simulink model "V3_2_MatlabFn_UnitTest"  (R2017b)
settings: Solver=VariableStepAuto  StartTime=0.0  StopTime=.5  MaxStep=1e-4  RelTol=1e-3
libraries: simulink x9, dspswit3 x1, powerlib x1
settings Model: Creator=Manu Krishnan  LastModifiedBy=Manu Krishnan

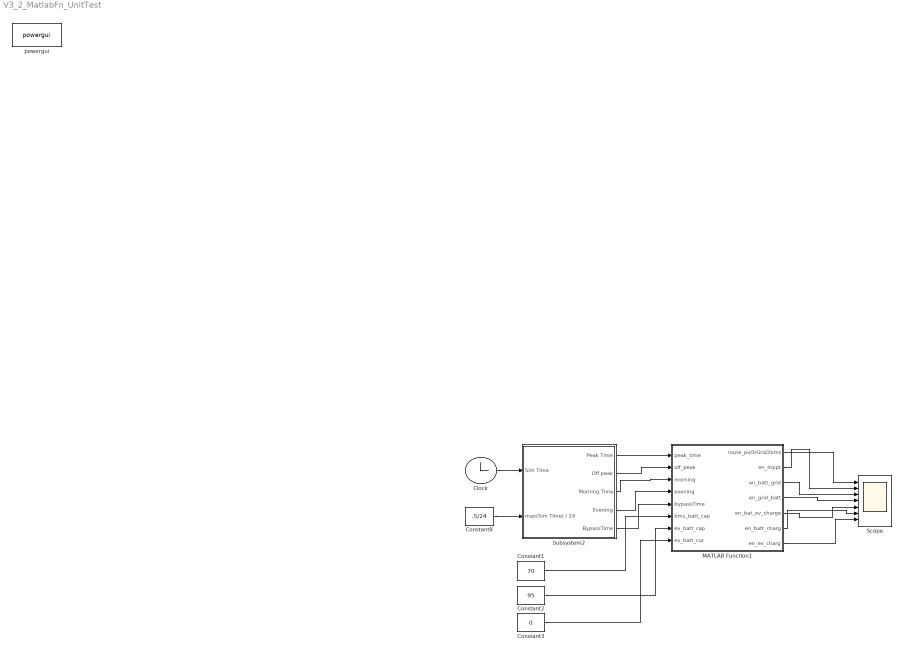
== system V3_2_MatlabFn_UnitTest ==
  Clock : Clock
  Constant1 : Constant  Value=70  VectorParams1D=off
  Constant2 : Constant  Value=95  VectorParams1D=off
  Constant3 : Constant  Value=0  VectorParams1D=off
  Constant8 : Constant  Value=.5/24  VectorParams1D=off
  MATLAB Function1 : MATLAB Function  TreatAsAtomicUnit=on
  Scope : Scope  NumInputPorts=7
  Subsystem2 : Subsystem
  powergui : powerlib/powergui  Priority=1  SimulationMode=Continuous  SampleTime=50e-6  frequency=60  Iterations=50  frequencyindice=0  Pbase=100e6  ErrMax=1e-4  UnitsV=kV  UnitsW=MW  buscounter=0  FunctionMessages=off  echomessages=off  EnableUseOfTLC=off  CurrentSourceSwitches=off  DisableSnubberDevices=off  DisableRonSwitches=off  DisableVfSwitches=off  DisplayEquations=off  SolverType=Tustin/Backward Euler (TBE)  Interpol=off  ExternalGateDelay=off  methode=off  Ts=100  x0status=blocks  SPID=on  SwTol=0  HookPort=off  RestoreLinks=warning  ResistiveCurrentMeasurement=off  Frange=[0:2:500]  Ylog=off  Xlog=on  ShowGrid=off  save=off  variable=ZData  structure=0  ZoomFFT=off  StartTime=0.0  cycles=1  DisplayStyle=1  fundamental=60  FreqAxis=off  MaxFrequency=1000  frequencyindicesteady=1  RmsSteady=1  display=off
  wires:
  Clock/1 -> Subsystem2/1(Sim Time)
  Constant8/1 -> Subsystem2/2(max(Sim Time) / 24)
  Subsystem2/1(Peak Time) -> MATLAB Function1/1(peak_time)
  Subsystem2/2(Off peak) -> MATLAB Function1/2(off_peak)
  Subsystem2/3(Morning Time) -> MATLAB Function1/3(morning)
  Subsystem2/4(Evening) -> MATLAB Function1/4(evening)
  Subsystem2/5(BypassTime) -> MATLAB Function1/5(bypassTime)
  MATLAB Function1/2(en_mppt) -> Scope/2
  MATLAB Function1/3(en_batt_grid) -> Scope/3
  MATLAB Function1/7(en_ev_charg) -> Scope/7
  MATLAB Function1/6(en_batt_charg) -> Scope/6
  MATLAB Function1/1(route_pvOrGrid2bms) -> Scope/1
  MATLAB Function1/5(en_bat_ev_charge) -> Scope/5
  MATLAB Function1/4(en_grid_batt) -> Scope/4
  Constant1/1 -> MATLAB Function1/6(bms_batt_cap)
  Constant2/1 -> MATLAB Function1/7(ev_batt_cap)
  Constant3/1 -> MATLAB Function1/8(ev_batt_cur)

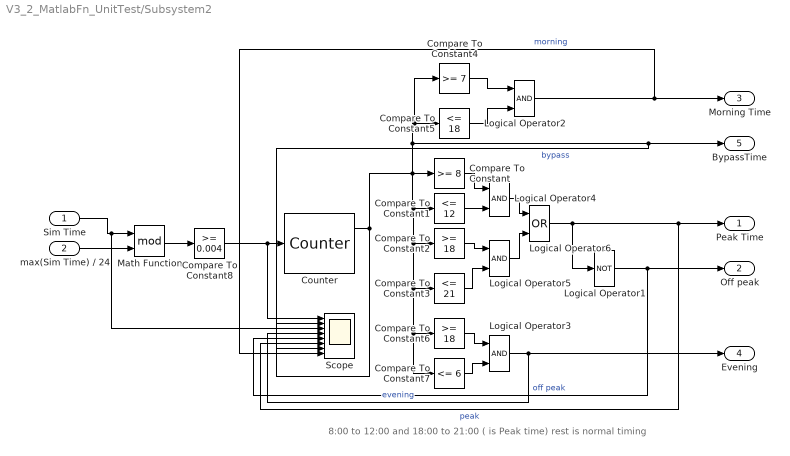
== system V3_2_MatlabFn_UnitTest/Subsystem2 ==
  note: 8:00 to 12:00 and 18:00 to 21:00 ( is Peak time)
      | rest is normal timing
  Sim Time : Inport
  max(Sim Time) / 24 : Inport  Port=2
  Compare To Constant : simulink/Logic and Bit Operations/Compare To Constant  relop=>=  const=8  OutDataTypeStr=boolean  ZeroCross=off
  Compare To Constant1 : simulink/Logic and Bit Operations/Compare To Constant  relop=<=  const=12  OutDataTypeStr=boolean  ZeroCross=off
  Compare To Constant2 : simulink/Logic and Bit Operations/Compare To Constant  relop=>=  const=18  OutDataTypeStr=boolean  ZeroCross=off
  Compare To Constant3 : simulink/Logic and Bit Operations/Compare To Constant  relop=<=  const=21  OutDataTypeStr=boolean  ZeroCross=off
  Compare To Constant4 : simulink/Logic and Bit Operations/Compare To Constant  relop=>=  const=7  OutDataTypeStr=boolean  ZeroCross=off
  Compare To Constant5 : simulink/Logic and Bit Operations/Compare To Constant  relop=<=  const=18  OutDataTypeStr=boolean  ZeroCross=off
  Compare To Constant6 : simulink/Logic and Bit Operations/Compare To Constant  relop=>=  const=18  OutDataTypeStr=boolean  ZeroCross=off
  Compare To Constant7 : simulink/Logic and Bit Operations/Compare To Constant  relop=<=  const=6  OutDataTypeStr=boolean  ZeroCross=off
  Compare To Constant8 : simulink/Logic and Bit Operations/Compare To Constant  relop=>=  const=0.004  OutDataTypeStr=boolean  ZeroCross=off
  Counter : dspswit3/Counter  Direction=Up  CountEvent=Falling edge  CounterSize=User defined  MaxCount=24  InitialCount=0  Output=Count and Hit  HitValue=24  ResetInput=off  SamplesPerFrame=1  Ts=1  CntDtype=int8  HitDtype=Logical
  Logical Operator1 : Logic  Operator=NOT  AllPortsSameDT=off  OutDataTypeStr=boolean
  Logical Operator{2..5} (4 alike) : Logic  AllPortsSameDT=off  OutDataTypeStr=boolean
  Logical Operator6 : Logic  Operator=OR  AllPortsSameDT=off  OutDataTypeStr=boolean
  Math Function : Math  Operator=mod  SaturateOnIntegerOverflow=on
  Scope : Scope  NumInputPorts=8
  Peak Time : Outport
  Off peak : Outport  Port=2
  Morning Time : Outport  Port=3
  Evening : Outport  Port=4
  BypassTime : Outport  Port=5
  wires:
  Sim Time/1 -> Scope/3, Math Function/1
  Logical Operator5/1 -> Logical Operator6/2
  Logical Operator4/1 -> Logical Operator6/1
  Compare To Constant1/1 -> Logical Operator4/2
  Compare To Constant3/1 -> Logical Operator5/2
  Compare To Constant/1 -> Logical Operator4/1
  Logical Operator6/1 -> Logical Operator1/1, Scope/6, Peak Time/1  "peak"
  Math Function/1 -> Compare To Constant8/1
  Compare To Constant2/1 -> Logical Operator5/1
  Logical Operator1/1 -> Scope/5, Off peak/1  "off peak"
  Compare To Constant4/1 -> Logical Operator2/1
  Compare To Constant5/1 -> Logical Operator2/2
  Logical Operator2/1 -> Scope/8, Morning Time/1  "morning"
  Compare To Constant6/1 -> Logical Operator3/1
  Compare To Constant7/1 -> Logical Operator3/2
  Logical Operator3/1 -> Scope/4, Evening/1  "evening"
  max(Sim Time) / 24/1 -> Math Function/2
  Compare To Constant8/1 -> Scope/1, Counter/1
  Counter/1 -> Scope/2, Scope/7, BypassTime/1, Compare To Constant5/1, Compare To Constant4/1, Compare To Constant7/1, Compare To Constant6/1, Compare To Constant3/1, Compare To Constant2/1, Compare To Constant1/1, Compare To Constant/1  "bypass"

== matlab function V3_2_MatlabFn_UnitTest/MATLAB Function1 ==
  data: route_pvOrGrid2bms output; en_mppt output; en_batt_grid output; en_grid_batt output; en_bat_ev_charge output; en_batt_charg output; en_ev_charg output; peak_time input; off_peak input; morning input; evening input; bypassTime input; bms_batt_cap input; ev_batt_cap input; ev_batt_cur input
function [route_pvOrGrid2bms, en_mppt,en_batt_grid, en_grid_batt, en_bat_ev_charge, en_batt_charg,en_ev_charg]= Automate(peak_time,off_peak,morning,evening,bypassTime,bms_batt_cap,ev_batt_cap,ev_batt_cur)
from_grid = 2;
from_solar =1;
if(ev_batt_cur < 1)
    carPresent = 0;
else
    carPresent =1;
end

% MODE 1 
% PV to battery
%---------------------------------------------------------------------------------------
%Time	        |Speicific Time	|EV 	             |BatteryBank Capacity	|EV battery
%---------------------------------------------------------------------------------------
%Morning 	    |Off peak	    |Not present         |<80%	                |>90%
%---------------------------------------------------------------------------------------
if  (off_peak &&   carPresent==0 && bms_batt_cap < 80 && ev_batt_cap > 90)
    en_batt_charg =1;
    en_mppt =1;
    route_pvOrGrid2bms =from_solar;
    en_batt_grid =0;
    en_grid_batt =0;
    en_ev_charg =0;
    en_bat_ev_charge =0;
%####################################################################################### 
% MODE 2
% PV to Electric Vehicle 
%---------------------------------------------------------------------------------------
%Time	        |Speicific Time	|EV 	             |BatteryBank Capacity	|EV battery
%---------------------------------------------------------------------------------------
%Morning 	    |Off peak	    |Present             |NA	                |<90%
% 
%---------------------------------------------------------------------------------------
elseif (off_peak && morning &&  carPresent==1 && ev_batt_cap < 90)
    en_batt_charg =1;
    en_mppt =1;
    route_pvOrGrid2bms =from_solar;
    en_batt_grid =0;
    en_grid_batt =0;
    en_ev_charg =0;
    en_bat_ev_charge =0;
%#######################################################################################    
% MODE 3
% Battery Bank to EV 
%---------------------------------------------------------------------------------------
%Time	        |Speicific Time	|EV 	             |BatteryBank Capacity	|EV battery
%---------------------------------------------------------------------------------------
%Evening	    |18:00 to 21:00	|Present	         | >30%                 |	<90%
%---------------------------------------------------------------------------------------
elseif (peak_time && evening &&  carPresent==1 && bms_batt_cap >30 && ev_batt_cap < 90)
    en_batt_charg =1;
    en_mppt =1;
    route_pvOrGrid2bms =from_grid;
    en_batt_grid =0;
    en_grid_batt =0;
    en_ev_charg =1;
    en_bat_ev_charge =1;   
%#######################################################################################  
% MODE 4
% AC grid to EV
%---------------------------------------------------------------------------------------
%Time	        |Speicific Time	|EV 	             |BatteryBank Capacity	|EV battery
%---------------------------------------------------------------------------------------
%Morning 	    |Off peak	    |Not present         |<80%	                |>90%
%---------------------------------------------------------------------------------------
elseif (off_peak && morning &&   carPresent==0 && bms_batt_cap <80 && ev_batt_cap < 90)
    en_batt_charg =1;
    en_mppt =1;
    route_pvOrGrid2bms =from_grid;
    en_batt_grid =0;
    en_grid_batt =0;
    en_ev_charg =1;
    en_bat_ev_charge =0;
%#######################################################################################  
% MODE 5
%PV to AC grid 
%---------------------------------------------------------------------------------------
%Time	        |Speicific Time	|EV 	             |BatteryBank Capacity	|EV battery
%---------------------------------------------------------------------------------------
%Morning 	    |NA	            |Not present         |<80%	                |>90%
%---------------------------------------------------------------------------------------
elseif (morning &&  bms_batt_cap >90 && carPresent==0  && ev_batt_cap > 90)
    en_batt_charg =1;
    en_mppt =1;
    route_pvOrGrid2bms =from_grid;
    en_batt_grid =0;
    en_grid_batt =0;
    en_ev_charg =0;
    en_bat_ev_charge =0;
else
    en_batt_charg =0;
    en_mppt =0;
    route_pvOrGrid2bms =from_grid;
    en_batt_grid =0;
    en_grid_batt =0;
    en_ev_charg =0;
    en_bat_ev_charge =0;

end
